simulink model "TP02_MyModel"  (R2023a)
settings: Solver=VariableStepAuto  StartTime=0.0  StopTime=10.0  RelTol=1e-3
undefined symbols (not defined in the file): g, K, l, u0, x0, xe
settings Model: Creator=crt4254  LastModifiedBy=crt4254

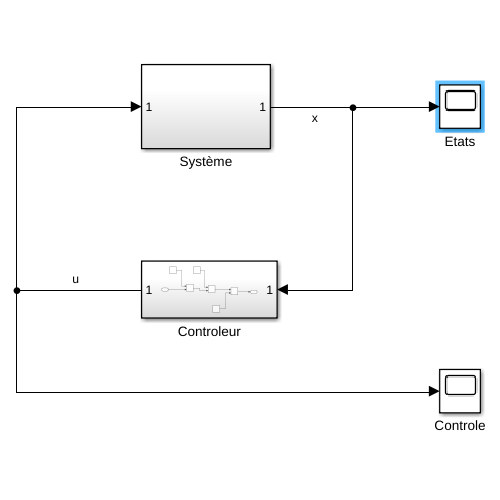
[thumbnail: Simulink's stored preview of the top-level diagram]
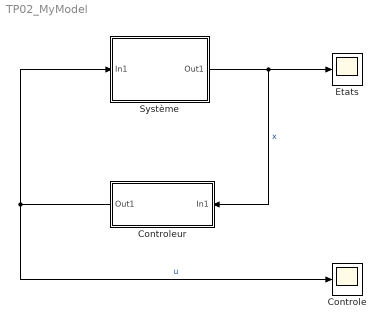
== system TP02_MyModel ==
  Controle : Scope
  Controleur : Subsystem
  Etats : Scope
  Système : Subsystem
  wires:
  Système/1(Out1) -> Controleur/1(In1), Etats/1  "x"
  Controleur/1(Out1) -> Controle/1, Système/1(In1)  "u"

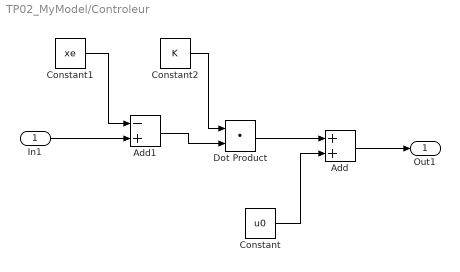
== system TP02_MyModel/Controleur ==
  In1 : Inport
  Add : Sum
  Add1 : Sum  Inputs=-+
  Constant : Constant  Value=u0
  Constant1 : Constant  Value=xe
  Constant2 : Constant  Value=K
  Dot Product : DotProduct  OutDataTypeStr=Inherit: Inherit via internal rule
  Out1 : Outport
  wires:
  Constant/1 -> Add/2
  In1/1 -> Add1/2
  Constant1/1 -> Add1/1
  Dot Product/1 -> Add/1
  Add1/1 -> Dot Product/2
  Constant2/1 -> Dot Product/1
  Add/1 -> Out1/1

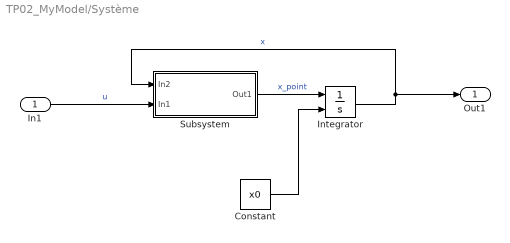
== system TP02_MyModel/Système ==
  In1 : Inport
  Constant : Constant  Value=x0
  Integrator : Integrator  InitialConditionSource=external  InitialCondition=x0
  Subsystem : Subsystem
  Out1 : Outport
  wires:
  Integrator/1 -> Subsystem/1(In2), Out1/1  "x"
  In1/1 -> Subsystem/2(In1)  "u"
  Subsystem/1(Out1) -> Integrator/1  "x_point"
  Constant/1 -> Integrator/2

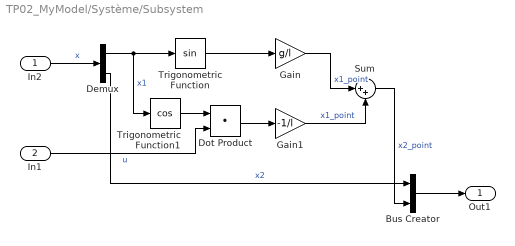
== system TP02_MyModel/Système/Subsystem ==
  In2 : Inport
  In1 : Inport  Port=2
  Bus Creator : BusCreator  Inputs=2
  Demux : Demux  Outputs=2
  Dot Product : DotProduct  OutDataTypeStr=Inherit: Inherit via internal rule
  Gain : Gain  Gain=g/l
  Gain1 : Gain  Gain=-1/l
  Sum : Sum  Inputs=|++
  Trigonometric Function : Trigonometry
  Trigonometric Function1 : Trigonometry  Operator=cos
  Out1 : Outport
  wires:
  In2/1 -> Demux/1  "x"
  Demux/1 -> Trigonometric Function1/1, Trigonometric Function/1  "x1"
  Trigonometric Function/1 -> Gain/1
  Bus Creator/1 -> Out1/1
  Trigonometric Function1/1 -> Dot Product/1
  Dot Product/1 -> Gain1/1
  In1/1 -> Dot Product/2  "u"
  Gain/1 -> Sum/1  "x1_point"
  Gain1/1 -> Sum/2  "x1_point"
  Sum/1 -> Bus Creator/2  "x2_point"
  Demux/2 -> Bus Creator/1  "x2"
